simulink model "Controller"  (R2022b)
settings: Solver=ode4  StartTime=0.0  StopTime=40  FixedStep=0.00001  RelTol=1e-3
settings Model: Creator=Sahil Gaurkar  LastModifiedBy=Sahil Gaurkar

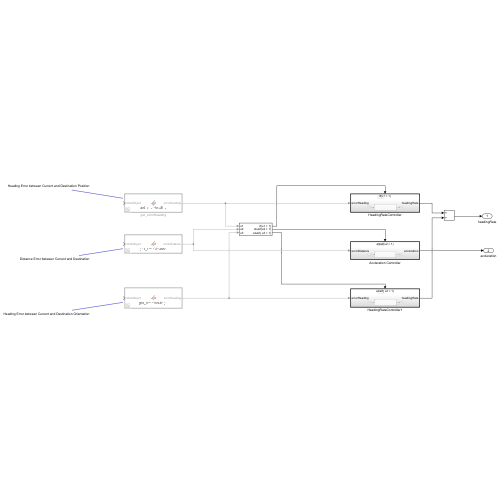
[thumbnail: Simulink's stored preview of the top-level diagram]
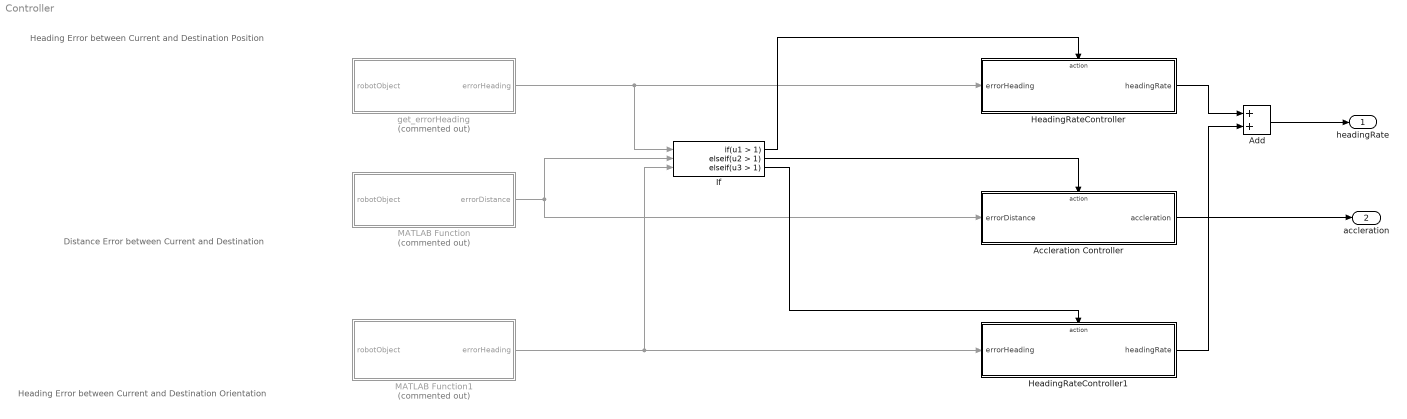
== system Controller ==
  note: Heading Error between Current and Destination Orientation
  note: Heading Error between Current and Destination Position
  note: Distance Error between Current and Destination
  Accleration Controller : Subsystem  TreatAsAtomicUnit=on
  Add : Sum
  HeadingRateController : Subsystem  TreatAsAtomicUnit=on
  HeadingRateController1 : Subsystem  TreatAsAtomicUnit=on
  If : If  NumInputs=3  IfExpression=u1 > 1  ElseIfExpressions=u2 > 1, u3 > 1  ShowElse=off
  MATLAB Function : MATLAB Function  Commented=on  TreatAsAtomicUnit=on
  MATLAB Function1 : MATLAB Function  Commented=on  TreatAsAtomicUnit=on
  get_errorHeading : MATLAB Function  Commented=on  TreatAsAtomicUnit=on
  headingRate : Outport
  accleration : Outport  Port=2
  wires:
  get_errorHeading/1(errorHeading) -> If/1, HeadingRateController/1(errorHeading)
  MATLAB Function/1(errorDistance) -> Accleration Controller/1(errorDistance), If/2
  MATLAB Function1/1(errorHeading) -> If/3, HeadingRateController1/1(errorHeading)
  HeadingRateController/1(headingRate) -> Add/1
  Add/1 -> headingRate/1
  If/2 -> Accleration Controller/Action
  If/1 -> HeadingRateController/Action
  If/3 -> HeadingRateController1/Action
  HeadingRateController1/1(headingRate) -> Add/2
  Accleration Controller/1(accleration) -> accleration/1

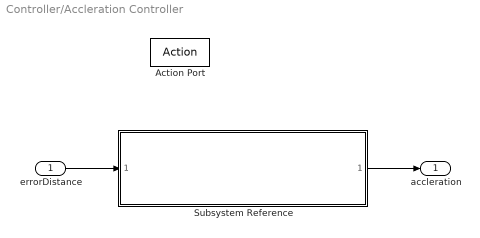
== system Controller/Accleration Controller ==
  errorDistance : Inport
  Action Port : ActionPort  ActionPortLabel=elseif(u2 > 1)
  Subsystem Reference : Subsystem  ReferencedSubsystem=AcclerationController
  accleration : Outport
  wires:
  errorDistance/1 -> Subsystem Reference/1
  Subsystem Reference/1 -> accleration/1

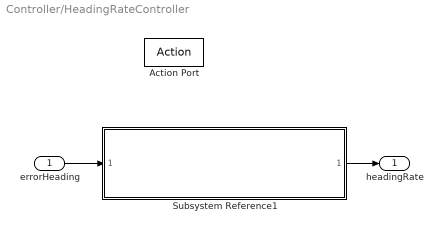
== system Controller/HeadingRateController ==
  errorHeading : Inport
  Action Port : ActionPort  ActionPortLabel=if(u1 > 1)
  Subsystem Reference1 : Subsystem  ReferencedSubsystem=HeadingRateController
  headingRate : Outport
  wires:
  errorHeading/1 -> Subsystem Reference1/1
  Subsystem Reference1/1 -> headingRate/1

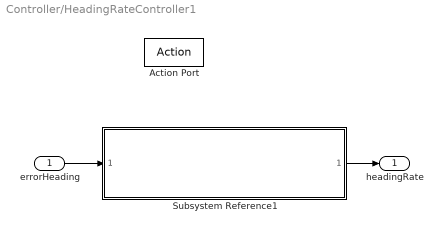
== system Controller/HeadingRateController1 ==
  errorHeading : Inport
  Action Port : ActionPort  ActionPortLabel=elseif( u3 > 1)
  Subsystem Reference1 : Subsystem  ReferencedSubsystem=HeadingRateController
  headingRate : Outport
  wires:
  errorHeading/1 -> Subsystem Reference1/1
  Subsystem Reference1/1 -> headingRate/1

== matlab function Controller/MATLAB Function ==
  data: robotObject input; errorDistance output
function errorDistance = get_errorDistance(robotObject)

errorDistance = pdist2(robotObject.destinationPose(1:2), robotObject.currentPose(1:2), 'euclidean');

end

== matlab function Controller/MATLAB Function1 ==
  data: robotObject input; errorHeading output
function errorHeading = get_errorHeading1(robotObject)

errorHeading = robotObject.destinationPose(3) - robotObject.currentPose(3);

end

== matlab function Controller/get_errorHeading ==
  data: robotObject input; errorHeading output
function errorHeading = get_errorHeading(robotObject)
errorHeading = atan2d(robotObject.destinationPose(2) - robotObject.currentPose(2), robotObject.destinationPose(1) - robotObject.currentPose(1)) - robotObject.currentPose(3);
end
